simulink model "MotorSlider_Sim_controlled"  (R2026a)
settings: Solver=FixedStepAuto  StopTime=1  FixedStep=0.001
values from neighbouring files (symbols this model uses):
  den_C = [1, -1]    [Task2_run.m]
  num_C = [q0, q1]    [Task2_run.m]
libraries: simulink x1
settings Model: Creator=lin-t  LastModifiedBy=adam
settings SimscapeCC: SimscapeNominalValues="[{\"value\":\"1\",\"unit\":\"A\"},{\"value\":\"1\",\"unit\":\"bar\"},{\"value\":\"1\",\"unit\":\"cm^2\"},{\"value\":\"1\",\"unit\":\"cm^3/s\"},{\"value\":\"1\",\"unit\":\"kJ/kg\"},{\"value\":\"1\",\"unit\":\"kW\"},{\"value\":\"1\",\"unit\":\"l\"},{\"value\":\"1\",\"unit\":\"N\"},{\"value\":\"1\",\"unit\":\"N*m\"},{\"value\":\"1\",\"unit\":\"V\"}]"  SimscapeLogType=none  SimscapeLogDataHistory=5000.0

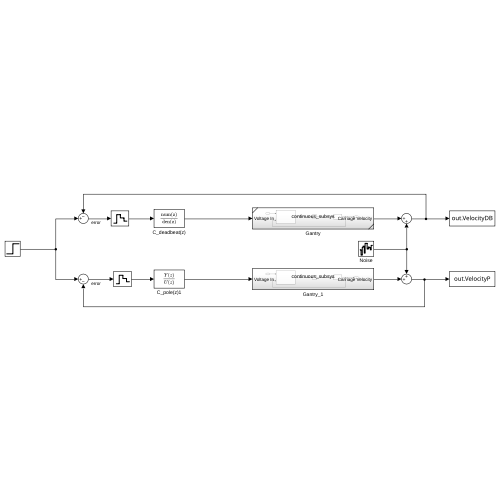
[thumbnail: Simulink's stored preview of the top-level diagram]
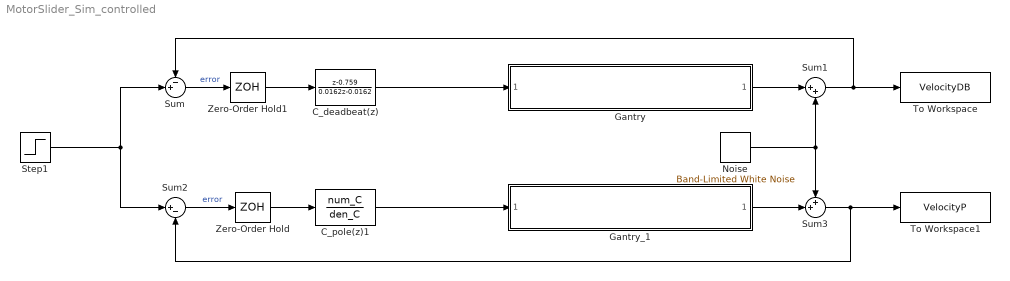
== system MotorSlider_Sim_controlled ==
  C_deadbeat(z) : DiscreteTransferFcn  Numerator=[1 -0.759]  Denominator=[0.0162 -0.0162]
  C_pole(z)1 : DiscreteTransferFcn  Numerator=num_C  Denominator=den_C
  Gantry : Subsystem  ReferencedSubsystem=continuous_subsys
  Gantry_1 : Subsystem  ReferencedSubsystem=continuous_subsys
  Noise : simulink/Sources/Band-Limited White Noise  Cov=noise_power  Ts=0.01  seed=[23341]
  Step1 : Step  Time=.3  FinalValue=velocityStep  SampleTime=0
  Sum : Sum  Inputs=-+|
  Sum1 : Sum  Inputs=|++
  Sum2 : Sum  Inputs=|+-
  Sum3 : Sum  Inputs=++|
  To Workspace : ToWorkspace  VariableName=VelocityDB  SaveFormat=Timeseries  SampleTime=-1
  To Workspace1 : ToWorkspace  VariableName=VelocityP  SaveFormat=Timeseries  SampleTime=-1
  Zero-Order Hold : ZeroOrderHold  SampleTime=0.02
  Zero-Order Hold1 : ZeroOrderHold  SampleTime=0.02
  wires:
  Sum1/1 -> To Workspace/1, Sum/1
  Gantry/1 -> Sum1/1
  Noise/1 -> Sum1/2, Sum3/1
  Step1/1 -> Sum2/1, Sum/2
  Sum3/1 -> Sum2/2, To Workspace1/1
  C_pole(z)1/1 -> Gantry_1/1
  Zero-Order Hold/1 -> C_pole(z)1/1
  Sum2/1 -> Zero-Order Hold/1  "error"
  Sum/1 -> Zero-Order Hold1/1  "error"
  Zero-Order Hold1/1 -> C_deadbeat(z)/1
  Gantry_1/1 -> Sum3/2
  C_deadbeat(z)/1 -> Gantry/1
